simulink model "muscle_1_PS3"  (R2024b)
settings: Solver=FixedStepAuto  StartTime=0.0  StopTime=2.5  FixedStep=0.00005  RelTol=1e-3
values from neighbouring files (symbols this model uses):
  Fmax_VAS = 6000    [muscle_1_params.m]    (also in problem_1ab.m; problem_1c.m)
  K = 5    [muscle_1_params.m]    (also in problem_1ab.m; problem_1c.m)
  lopt_VAS = 0.08    [muscle_1_params.m]    (also in problem_1ab.m; problem_1c.m)
  N = 1.5    [muscle_1_params.m]    (also in problem_1ab.m; problem_1c.m)
  preA = 0.01    [muscle_1_params.m]    (also in problem_1ab.m; problem_1c.m)
  tau_ecc = 0.01    [muscle_1_params.m]    (also in problem_1ab.m; problem_1c.m)
  vmax_VAS = -12 * lopt_VAS    (= -0.96)    [muscle_1_params.m]    (also in problem_1ab.m = 0.96; problem_1c.m)
  w = 0.56    [muscle_1_params.m]    (also in problem_1ab.m; problem_1c.m)
undefined symbols (not defined in the file or in its folder): mass
settings Model: Creator=hgeyer  LastModifiedBy=gnastacast
settings SolverCC: EnableFixedStepZeroCrossing=on

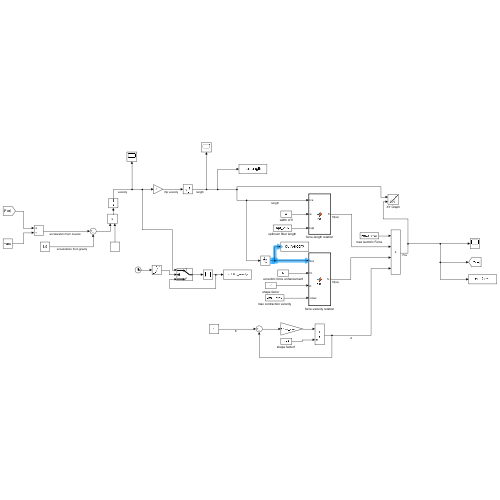
[thumbnail: Simulink's stored preview of the top-level diagram]
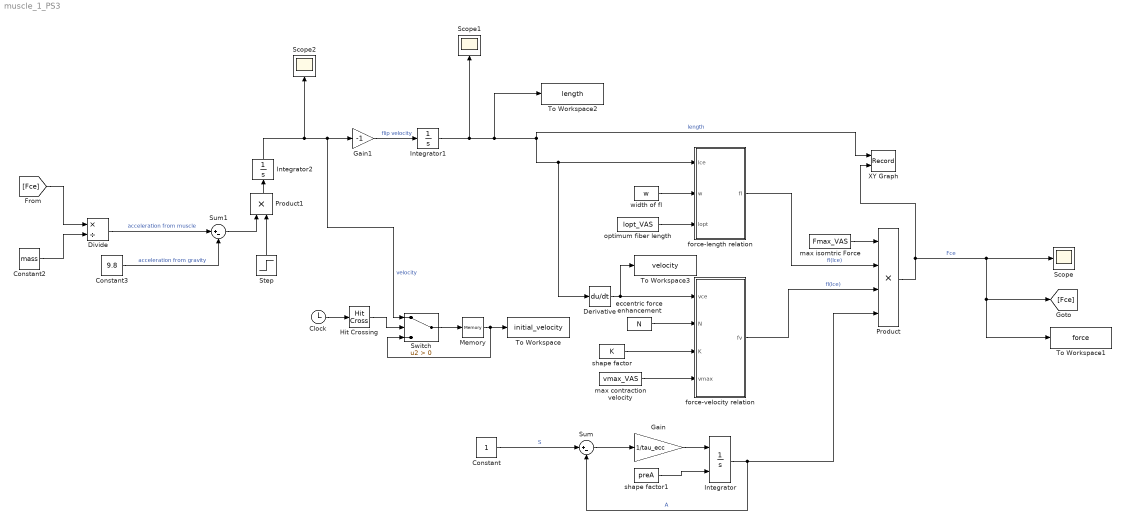
== system muscle_1_PS3 ==
  Clock : Clock
  Constant : Constant
  Constant2 : Constant  Value=mass
  Constant3 : Constant  Value=9.8
  Derivative : Derivative
  Divide : Product  Inputs=*/
  Gain : Gain  Gain=1/tau_ecc
  Gain1 : Gain  Gain=-1
  Hit Crossing : HitCross  HitCrossingOffset=1.01  HitCrossingDirection=rising
  Integrator : Integrator  InitialConditionSource=external
  Integrator1 : Integrator  InitialCondition=lopt_VAS  LimitOutput=on  UpperSaturationLimit=2*lopt_VAS  LowerSaturationLimit=0.5*lopt_VAS
  Integrator2 : Integrator
  Memory : Memory
  Product : Product  Inputs=4
  Product1 : Product
  Scope : Scope
  Scope1 : Scope
  Scope2 : Scope
  Step : Step  SampleTime=0
  Sum : Sum  Inputs=|+-
  Sum1 : Sum  Inputs=|+-
  Switch : Switch  Criteria=u2 > Threshold  SaturateOnIntegerOverflow=off  InputSameDT=off
  To Workspace : ToWorkspace  VariableName=initial_velocity  SampleTime=-1
      settings: MaxDataPoints=1
  To Workspace1 : ToWorkspace  VariableName=force  SaveFormat=Timeseries  SampleTime=-1
  To Workspace2 : ToWorkspace  VariableName=length  SaveFormat=Timeseries  SampleTime=-1
  To Workspace3 : ToWorkspace  VariableName=velocity  SaveFormat=Timeseries  SampleTime=-1
  XY Graph : Record  FileSettingsInternal="{\"entries\":[{\"content\":{\"excelSettings\":{\"content\":{},\"type\":\"Streamout.ExcelSettings\"}},\"type\":\"Streamout.FileSettingStorage\",\"uuid\":\"\"}],\"packageUris\":[\"http:\\/\\/schema.mathworks.com\\/mf0\\/streamout_blocks\\/R2020a\"],\"version\":\"1.0\"}"  Layout=[1 1]  SignalsInternal="{\"entries\":[{\"content\":{\"signals\":[{\"content\":{\"blockPath\":[],\"dimensions\":[1],\"domain\":\"\",\"lineColor\":\"#a2142f\",\"plots\":[ 1 ],\"port\":1,\"sid\":[\"\"],\"signalID\":1,\"signalName\":\"length\"},\"type\":\"RecordBlkView.Signal\",\"uuid\":\"\"},{\"content\":{\"blockPath\":[],\"dimensions\":[1],\"domain\":\"\",\"lineColor\":\"#139fff\",\"plots\":[ 1 ],\"port\":2,\"sid\":[\"\"],\"signalID\":2,\"signalName\":\"Fce\"},\"type\":\"RecordBlkView.Signal\",\"uuid\":\"\"}]},\"type\":\"RecordBlkView.InputSignals\",\"uuid\":\"\"}],\"packageUris\":[\"http:\\/\\/schema.mathworks.com\\/mf0\\/streamout_blocks\\/R2020a\"],\"version\":\"1.0\"}"  VisualizationBindings="{\"xyplotplugin\":{\"info\":[{\"series\":[{\"bindingParametersList\":[{\"parameter\":\"X-Axis\",\"signalID\":1,\"signalName\":\"length\"},{\"parameter\":\"Y-Axis\",\"signalID\":2,\"signalName\":\"Fce\"}],\"seriesID\":0}],\"subplotID\":1}]}}"  CompatibilityTag=XY
  eccentric force enhancement : Constant  Value=N
  force-length relation : MATLAB Function  TreatAsAtomicUnit=on
  force-velocity relation : MATLAB Function  TreatAsAtomicUnit=on
  max contraction velocity : Constant  Value=vmax_VAS
  max isomtric Force : Constant  Value=Fmax_VAS
  optimum fiber length : Constant  Value=lopt_VAS
  shape factor : Constant  Value=K
  shape factor1 : Constant  Value=preA
  width of fl : Constant  Value=w
  wires:
  width of fl/1 -> force-length relation/2(w)
  optimum fiber length/1 -> force-length relation/3(lopt)
  eccentric force enhancement/1 -> force-velocity relation/2(N)
  max contraction velocity/1 -> force-velocity relation/4(vmax)
  shape factor/1 -> force-velocity relation/3(K)
  force-velocity relation/1(fv) -> Product/3  "fl(lce)"
  force-length relation/1(fl) -> Product/2  "fl(lce)"
  max isomtric Force/1 -> Product/1
  Integrator/1 -> Product/4, Sum/2  "A"
  Derivative/1 -> To Workspace3/1, force-velocity relation/1(vce)
  Product/1 -> XY Graph/2, To Workspace1/1, [Fce], Scope/1  "Fce"
  shape factor1/1 -> Integrator/2
  Gain/1 -> Integrator/1
  Sum/1 -> Gain/1
  Constant/1 -> Sum/1  "S"
  Integrator1/1 -> To Workspace2/1, Derivative/1, force-length relation/1(lce), XY Graph/1, Scope1/1  "length"
  Integrator2/1 -> Switch/1, Gain1/1, Scope2/1  "velocity"
  [Fce] -> Divide/1
  Constant2/1 -> Divide/2
  Divide/1 -> Sum1/1  "acceleration from muscle"
  Step/1 -> Product1/2
  Product1/1 -> Integrator2/1
  Gain1/1 -> Integrator1/1  "flip velocity"
  Sum1/1 -> Product1/1
  Constant3/1 -> Sum1/2  "acceleration from gravity"
  Switch/1 -> Memory/1
  Memory/1 -> Switch/3, To Workspace/1
  Clock/1 -> Hit Crossing/1
  Hit Crossing/1 -> Switch/2

== matlab function muscle_1_PS3/force-velocity relation ==
  data: vce input; fv output; N input; K input; vmax input
function fv = fcn(vce, N, K, vmax)

if vce <= 0  % concentric motion
    fv = (vmax - vce) / (vmax + K*vce);
else  % eccentric motion
    fv = N + (N-1) * (vmax + vce) / (7.56 * K * vce - vmax);
end

== matlab function muscle_1_PS3/force-length relation ==
  data: lce input; fl output; w input; lopt input
function fl = fcn(lce, w, lopt)


fl = exp(-(lce-lopt)^2 / (w * lopt)^2);
